simulink model "gm_DUALportRAMinterface_v3_vnl"  (R2024a)
settings: Solver=FixedStepDiscrete  StartTime=0.0  StopTime=0.1  RelTol=1e-3
undefined symbols (not defined in the file or in its folder): magnitude, Ts
libraries: hdlsllib x227, embmathops x6, simulink x2, hdlmdlgenlib x1, dsphdlxfrm2 x1
(part 5 of 6)

== system gm_DUALportRAMinterface_v3_vnl/PL/integration_block1/accumulator_scorer/64bitmsb_finder/8bit_PE7 ==
  D7 : Inport
  D6 : Inport  Port=2
  D5 : Inport  Port=3
  D4 : Inport  Port=4
  D3 : Inport  Port=5
  D2 : Inport  Port=6
  D1 : Inport  Port=7
  D0 : Inport  Port=8
  Add : Sum
  Bit Concat : hdlsllib/Logic and Bit Operations/Bit Concat  numInputs=3
  Constant2 : Constant  OutDataTypeStr=fixdt(0,4,0)  SampleTime=Ts
  Constant3 : Constant  Value=0  OutDataTypeStr=fixdt(0,4,0)  SampleTime=Ts
  Logical Operator{,10..16,22} (9 alike) : Logic  Operator=NOT  IconShape=distinctive  AllPortsSameDT=off  OutDataTypeStr=boolean
  Logical Operator1 : Logic  Operator=NAND  IconShape=distinctive  AllPortsSameDT=off  OutDataTypeStr=boolean
  Logical Operator{17..20} (4 alike) : Logic  Operator=OR  Inputs=4  IconShape=distinctive  AllPortsSameDT=off  OutDataTypeStr=boolean
  Logical Operator2 : Logic  Operator=NAND  Inputs=4  IconShape=distinctive  AllPortsSameDT=off  OutDataTypeStr=boolean
  Logical Operator21 : Logic  Operator=NAND  Inputs=3  IconShape=distinctive  AllPortsSameDT=off  OutDataTypeStr=boolean
  Logical Operator23 : Logic  IconShape=distinctive  AllPortsSameDT=off  OutDataTypeStr=boolean
  Logical Operator3 : Logic  Operator=NAND  Inputs=3  IconShape=distinctive  AllPortsSameDT=off  OutDataTypeStr=boolean
  Logical Operator4 : Logic  Inputs=3  IconShape=distinctive  AllPortsSameDT=off  OutDataTypeStr=boolean
  Logical Operator5 : Logic  Inputs=3  IconShape=distinctive  AllPortsSameDT=off  OutDataTypeStr=boolean
  Logical Operator6 : Logic  Inputs=4  IconShape=distinctive  AllPortsSameDT=off  OutDataTypeStr=boolean
  Logical Operator7 : Logic  Operator=NAND  Inputs=3  IconShape=distinctive  AllPortsSameDT=off  OutDataTypeStr=boolean
  Logical Operator8 : Logic  Operator=NAND  Inputs=4  IconShape=distinctive  AllPortsSameDT=off  OutDataTypeStr=boolean
  Logical Operator9 : Logic  Operator=NAND  Inputs=4  IconShape=distinctive  AllPortsSameDT=off  OutDataTypeStr=boolean
  Switch : Switch  Criteria=u2 > Threshold  SaturateOnIntegerOverflow=off  InputSameDT=off  OutDataTypeStr=Inherit: Same as first input
  data2 : Outport
  valid : Outport  Port=2
  wires:
  Logical Operator1/1 -> Logical Operator4/2, Logical Operator6/2, Logical Operator5/2, Logical Operator2/2, Logical Operator3/1, Logical Operator11/1
  Logical Operator2/1 -> Logical Operator6/4, Logical Operator8/2, Logical Operator7/2, Logical Operator13/1
  Logical Operator18/1 -> Bit Concat/2, Logical Operator20/3, Logical Operator21/2
  Logical Operator3/1 -> Logical Operator2/1, Logical Operator6/1, Logical Operator5/1, Logical Operator4/1, Logical Operator12/1
  Logical Operator13/1 -> Logical Operator17/4
  D4/1 -> Logical Operator2/4
  Logical Operator7/1 -> Logical Operator9/2, Logical Operator8/3, Logical Operator14/1
  Logical Operator/1 -> Logical Operator1/1, Logical Operator2/3, Logical Operator6/3, Logical Operator5/3, Logical Operator4/3, Logical Operator3/2, Logical Operator10/1
  Logical Operator12/1 -> Logical Operator17/3, Logical Operator19/2
  Logical Operator19/1 -> Logical Operator20/4, Logical Operator21/3, Bit Concat/3
  D3/1 -> Logical Operator7/3
  D7/1 -> Logical Operator/1
  Logical Operator15/1 -> Logical Operator18/4
  Logical Operator10/1 -> Logical Operator19/1, Logical Operator18/1, Logical Operator17/1
  Logical Operator14/1 -> Logical Operator18/3, Logical Operator19/4
  D5/1 -> Logical Operator3/3
  Logical Operator17/1 -> Logical Operator20/1, Logical Operator21/1, Bit Concat/1
  D2/1 -> Logical Operator8/4
  Logical Operator5/1 -> Logical Operator8/1
  D1/1 -> Logical Operator9/4
  Logical Operator4/1 -> Logical Operator7/1
  Logical Operator8/1 -> Logical Operator9/3, Logical Operator15/1
  Logical Operator6/1 -> Logical Operator9/1
  D6/1 -> Logical Operator1/2
  Logical Operator11/1 -> Logical Operator18/2, Logical Operator17/2
  Logical Operator16/1 -> Logical Operator19/3
  Logical Operator9/1 -> Logical Operator16/1
  D0/1 -> Logical Operator20/2
  Logical Operator20/1 -> valid/1, Logical Operator22/1
  Switch/1 -> Add/1
  Constant3/1 -> Switch/1
  Add/1 -> data2/1
  Bit Concat/1 -> Add/2
  Constant2/1 -> Switch/3
  Logical Operator21/1 -> Logical Operator23/1
  Logical Operator23/1 -> Switch/2
  Logical Operator22/1 -> Logical Operator23/2

== system gm_DUALportRAMinterface_v3_vnl/PL/integration_block1/accumulator_scorer/64bitmsb_finder/8bit_PE8 ==
  D7 : Inport
  D6 : Inport  Port=2
  D5 : Inport  Port=3
  D4 : Inport  Port=4
  D3 : Inport  Port=5
  D2 : Inport  Port=6
  D1 : Inport  Port=7
  D0 : Inport  Port=8
  Add : Sum
  Bit Concat : hdlsllib/Logic and Bit Operations/Bit Concat  numInputs=3
  Constant2 : Constant  OutDataTypeStr=fixdt(0,4,0)  SampleTime=Ts
  Constant3 : Constant  Value=0  OutDataTypeStr=fixdt(0,4,0)  SampleTime=Ts
  Logical Operator{,10..16,22} (9 alike) : Logic  Operator=NOT  IconShape=distinctive  AllPortsSameDT=off  OutDataTypeStr=boolean
  Logical Operator1 : Logic  Operator=NAND  IconShape=distinctive  AllPortsSameDT=off  OutDataTypeStr=boolean
  Logical Operator{17..20} (4 alike) : Logic  Operator=OR  Inputs=4  IconShape=distinctive  AllPortsSameDT=off  OutDataTypeStr=boolean
  Logical Operator2 : Logic  Operator=NAND  Inputs=4  IconShape=distinctive  AllPortsSameDT=off  OutDataTypeStr=boolean
  Logical Operator21 : Logic  Operator=NAND  Inputs=3  IconShape=distinctive  AllPortsSameDT=off  OutDataTypeStr=boolean
  Logical Operator23 : Logic  IconShape=distinctive  AllPortsSameDT=off  OutDataTypeStr=boolean
  Logical Operator3 : Logic  Operator=NAND  Inputs=3  IconShape=distinctive  AllPortsSameDT=off  OutDataTypeStr=boolean
  Logical Operator4 : Logic  Inputs=3  IconShape=distinctive  AllPortsSameDT=off  OutDataTypeStr=boolean
  Logical Operator5 : Logic  Inputs=3  IconShape=distinctive  AllPortsSameDT=off  OutDataTypeStr=boolean
  Logical Operator6 : Logic  Inputs=4  IconShape=distinctive  AllPortsSameDT=off  OutDataTypeStr=boolean
  Logical Operator7 : Logic  Operator=NAND  Inputs=3  IconShape=distinctive  AllPortsSameDT=off  OutDataTypeStr=boolean
  Logical Operator8 : Logic  Operator=NAND  Inputs=4  IconShape=distinctive  AllPortsSameDT=off  OutDataTypeStr=boolean
  Logical Operator9 : Logic  Operator=NAND  Inputs=4  IconShape=distinctive  AllPortsSameDT=off  OutDataTypeStr=boolean
  Switch : Switch  Criteria=u2 > Threshold  SaturateOnIntegerOverflow=off  InputSameDT=off  OutDataTypeStr=Inherit: Same as first input
  data2 : Outport
  valid : Outport  Port=2
  wires:
  Logical Operator22/1 -> Logical Operator23/2
  Logical Operator23/1 -> Switch/2
  Logical Operator21/1 -> Logical Operator23/1
  Constant2/1 -> Switch/3
  Bit Concat/1 -> Add/2
  Add/1 -> data2/1
  Constant3/1 -> Switch/1
  Switch/1 -> Add/1
  Logical Operator20/1 -> Logical Operator22/1, valid/1
  D0/1 -> Logical Operator20/2
  Logical Operator9/1 -> Logical Operator16/1
  Logical Operator16/1 -> Logical Operator19/3
  Logical Operator11/1 -> Logical Operator17/2, Logical Operator18/2
  D6/1 -> Logical Operator1/2
  Logical Operator6/1 -> Logical Operator9/1
  Logical Operator8/1 -> Logical Operator15/1, Logical Operator9/3
  Logical Operator4/1 -> Logical Operator7/1
  D1/1 -> Logical Operator9/4
  Logical Operator5/1 -> Logical Operator8/1
  D2/1 -> Logical Operator8/4
  Logical Operator17/1 -> Bit Concat/1, Logical Operator21/1, Logical Operator20/1
  D5/1 -> Logical Operator3/3
  Logical Operator14/1 -> Logical Operator19/4, Logical Operator18/3
  Logical Operator10/1 -> Logical Operator17/1, Logical Operator18/1, Logical Operator19/1
  Logical Operator15/1 -> Logical Operator18/4
  D7/1 -> Logical Operator/1
  D3/1 -> Logical Operator7/3
  Logical Operator19/1 -> Bit Concat/3, Logical Operator21/3, Logical Operator20/4
  Logical Operator12/1 -> Logical Operator19/2, Logical Operator17/3
  Logical Operator/1 -> Logical Operator10/1, Logical Operator3/2, Logical Operator4/3, Logical Operator5/3, Logical Operator6/3, Logical Operator2/3, Logical Operator1/1
  Logical Operator7/1 -> Logical Operator14/1, Logical Operator8/3, Logical Operator9/2
  D4/1 -> Logical Operator2/4
  Logical Operator13/1 -> Logical Operator17/4
  Logical Operator3/1 -> Logical Operator12/1, Logical Operator4/1, Logical Operator5/1, Logical Operator6/1, Logical Operator2/1
  Logical Operator18/1 -> Logical Operator21/2, Logical Operator20/3, Bit Concat/2
  Logical Operator2/1 -> Logical Operator13/1, Logical Operator7/2, Logical Operator8/2, Logical Operator6/4
  Logical Operator1/1 -> Logical Operator11/1, Logical Operator3/1, Logical Operator2/2, Logical Operator5/2, Logical Operator6/2, Logical Operator4/2

== system gm_DUALportRAMinterface_v3_vnl/PL/integration_block1/GA_main/coefficent_array/individual1/Subsystem ==
  reg_in : Inport
  enable : Inport  Port=2
  Delay : Delay  DelayLength=1  InitialCondition=0  SampleTime=Ts
  Switch : Switch  Criteria=u2 > Threshold  SaturateOnIntegerOverflow=off  InputSameDT=off
  reg_out : Outport
  wires:
  reg_in/1 -> Switch/1
  enable/1 -> Switch/2
  Switch/1 -> Delay/1
  Delay/1 -> Switch/3, reg_out/1

== system gm_DUALportRAMinterface_v3_vnl/PL/integration_block1/GA_main/coefficent_array/individual1/Subsystem1 ==
  reg_in : Inport
  enable : Inport  Port=2
  Delay : Delay  DelayLength=1  InitialCondition=0  SampleTime=Ts
  Switch : Switch  Criteria=u2 > Threshold  SaturateOnIntegerOverflow=off  InputSameDT=off
  reg_out : Outport
  wires:
  reg_in/1 -> Switch/1
  enable/1 -> Switch/2
  Switch/1 -> Delay/1
  Delay/1 -> Switch/3, reg_out/1

== system gm_DUALportRAMinterface_v3_vnl/PL/integration_block1/GA_main/coefficent_array/individual1/Subsystem2 ==
  reg_in : Inport
  enable : Inport  Port=2
  Delay : Delay  DelayLength=1  InitialCondition=0  SampleTime=Ts
  Switch : Switch  Criteria=u2 > Threshold  SaturateOnIntegerOverflow=off  InputSameDT=off
  reg_out : Outport
  wires:
  reg_in/1 -> Switch/1
  enable/1 -> Switch/2
  Switch/1 -> Delay/1
  Delay/1 -> Switch/3, reg_out/1

== system gm_DUALportRAMinterface_v3_vnl/PL/integration_block1/GA_main/coefficent_array/individual1/Subsystem3 ==
  reg_in : Inport
  enable : Inport  Port=2
  Delay : Delay  DelayLength=1  InitialCondition=0  SampleTime=Ts
  Switch : Switch  Criteria=u2 > Threshold  SaturateOnIntegerOverflow=off  InputSameDT=off
  reg_out : Outport
  wires:
  reg_in/1 -> Switch/1
  enable/1 -> Switch/2
  Switch/1 -> Delay/1
  Delay/1 -> Switch/3, reg_out/1

== system gm_DUALportRAMinterface_v3_vnl/PL/integration_block1/GA_main/coefficent_array/individual1/Subsystem4 ==
  reg_in : Inport
  enable : Inport  Port=2
  Delay : Delay  DelayLength=1  InitialCondition=0  SampleTime=Ts
  Switch : Switch  Criteria=u2 > Threshold  SaturateOnIntegerOverflow=off  InputSameDT=off
  reg_out : Outport
  wires:
  reg_in/1 -> Switch/1
  enable/1 -> Switch/2
  Switch/1 -> Delay/1
  Delay/1 -> Switch/3, reg_out/1

== system gm_DUALportRAMinterface_v3_vnl/PL/integration_block1/GA_main/coefficent_array/individual1/Subsystem5 ==
  reg_in : Inport
  enable : Inport  Port=2
  Delay : Delay  DelayLength=1  InitialCondition=0  SampleTime=Ts
  Switch : Switch  Criteria=u2 > Threshold  SaturateOnIntegerOverflow=off  InputSameDT=off
  reg_out : Outport
  wires:
  reg_in/1 -> Switch/1
  enable/1 -> Switch/2
  Switch/1 -> Delay/1
  Delay/1 -> Switch/3, reg_out/1

== system gm_DUALportRAMinterface_v3_vnl/PL/integration_block1/GA_main/coefficent_array/individual1/Subsystem6 ==
  reg_in : Inport
  enable : Inport  Port=2
  Delay : Delay  DelayLength=1  InitialCondition=0  SampleTime=Ts
  Switch : Switch  Criteria=u2 > Threshold  SaturateOnIntegerOverflow=off  InputSameDT=off
  reg_out : Outport
  wires:
  Delay/1 -> reg_out/1, Switch/3
  Switch/1 -> Delay/1
  enable/1 -> Switch/2
  reg_in/1 -> Switch/1

== system gm_DUALportRAMinterface_v3_vnl/PL/integration_block1/GA_main/coefficent_array/individual2/Subsystem ==
  reg_in : Inport
  enable : Inport  Port=2
  Delay : Delay  DelayLength=1  InitialCondition=0  SampleTime=Ts
  Switch : Switch  Criteria=u2 > Threshold  SaturateOnIntegerOverflow=off  InputSameDT=off
  reg_out : Outport
  wires:
  Delay/1 -> reg_out/1, Switch/3
  Switch/1 -> Delay/1
  enable/1 -> Switch/2
  reg_in/1 -> Switch/1

== system gm_DUALportRAMinterface_v3_vnl/PL/integration_block1/GA_main/coefficent_array/individual2/Subsystem1 ==
  reg_in : Inport
  enable : Inport  Port=2
  Delay : Delay  DelayLength=1  InitialCondition=0  SampleTime=Ts
  Switch : Switch  Criteria=u2 > Threshold  SaturateOnIntegerOverflow=off  InputSameDT=off
  reg_out : Outport
  wires:
  Delay/1 -> reg_out/1, Switch/3
  Switch/1 -> Delay/1
  enable/1 -> Switch/2
  reg_in/1 -> Switch/1

== system gm_DUALportRAMinterface_v3_vnl/PL/integration_block1/GA_main/coefficent_array/individual2/Subsystem2 ==
  reg_in : Inport
  enable : Inport  Port=2
  Delay : Delay  DelayLength=1  InitialCondition=0  SampleTime=Ts
  Switch : Switch  Criteria=u2 > Threshold  SaturateOnIntegerOverflow=off  InputSameDT=off
  reg_out : Outport
  wires:
  Delay/1 -> reg_out/1, Switch/3
  Switch/1 -> Delay/1
  enable/1 -> Switch/2
  reg_in/1 -> Switch/1

== system gm_DUALportRAMinterface_v3_vnl/PL/integration_block1/GA_main/coefficent_array/individual2/Subsystem3 ==
  reg_in : Inport
  enable : Inport  Port=2
  Delay : Delay  DelayLength=1  InitialCondition=0  SampleTime=Ts
  Switch : Switch  Criteria=u2 > Threshold  SaturateOnIntegerOverflow=off  InputSameDT=off
  reg_out : Outport
  wires:
  Delay/1 -> reg_out/1, Switch/3
  Switch/1 -> Delay/1
  enable/1 -> Switch/2
  reg_in/1 -> Switch/1

== system gm_DUALportRAMinterface_v3_vnl/PL/integration_block1/GA_main/coefficent_array/individual2/Subsystem4 ==
  reg_in : Inport
  enable : Inport  Port=2
  Delay : Delay  DelayLength=1  InitialCondition=0  SampleTime=Ts
  Switch : Switch  Criteria=u2 > Threshold  SaturateOnIntegerOverflow=off  InputSameDT=off
  reg_out : Outport
  wires:
  Delay/1 -> reg_out/1, Switch/3
  Switch/1 -> Delay/1
  enable/1 -> Switch/2
  reg_in/1 -> Switch/1

== system gm_DUALportRAMinterface_v3_vnl/PL/integration_block1/GA_main/coefficent_array/individual2/Subsystem5 ==
  reg_in : Inport
  enable : Inport  Port=2
  Delay : Delay  DelayLength=1  InitialCondition=0  SampleTime=Ts
  Switch : Switch  Criteria=u2 > Threshold  SaturateOnIntegerOverflow=off  InputSameDT=off
  reg_out : Outport
  wires:
  Delay/1 -> reg_out/1, Switch/3
  Switch/1 -> Delay/1
  enable/1 -> Switch/2
  reg_in/1 -> Switch/1

== system gm_DUALportRAMinterface_v3_vnl/PL/integration_block1/GA_main/coefficent_array/individual2/Subsystem6 ==
  reg_in : Inport
  enable : Inport  Port=2
  Delay : Delay  DelayLength=1  InitialCondition=0  SampleTime=Ts
  Switch : Switch  Criteria=u2 > Threshold  SaturateOnIntegerOverflow=off  InputSameDT=off
  reg_out : Outport
  wires:
  reg_in/1 -> Switch/1
  enable/1 -> Switch/2
  Switch/1 -> Delay/1
  Delay/1 -> Switch/3, reg_out/1

== system gm_DUALportRAMinterface_v3_vnl/PL/integration_block1/GA_main/coefficent_array/individual3/Subsystem ==
  reg_in : Inport
  enable : Inport  Port=2
  Delay : Delay  DelayLength=1  InitialCondition=0  SampleTime=Ts
  Switch : Switch  Criteria=u2 > Threshold  SaturateOnIntegerOverflow=off  InputSameDT=off
  reg_out : Outport
  wires:
  reg_in/1 -> Switch/1
  enable/1 -> Switch/2
  Switch/1 -> Delay/1
  Delay/1 -> Switch/3, reg_out/1

== system gm_DUALportRAMinterface_v3_vnl/PL/integration_block1/GA_main/coefficent_array/individual3/Subsystem1 ==
  reg_in : Inport
  enable : Inport  Port=2
  Delay : Delay  DelayLength=1  InitialCondition=0  SampleTime=Ts
  Switch : Switch  Criteria=u2 > Threshold  SaturateOnIntegerOverflow=off  InputSameDT=off
  reg_out : Outport
  wires:
  reg_in/1 -> Switch/1
  enable/1 -> Switch/2
  Switch/1 -> Delay/1
  Delay/1 -> Switch/3, reg_out/1

== system gm_DUALportRAMinterface_v3_vnl/PL/integration_block1/GA_main/coefficent_array/individual3/Subsystem2 ==
  reg_in : Inport
  enable : Inport  Port=2
  Delay : Delay  DelayLength=1  InitialCondition=0  SampleTime=Ts
  Switch : Switch  Criteria=u2 > Threshold  SaturateOnIntegerOverflow=off  InputSameDT=off
  reg_out : Outport
  wires:
  reg_in/1 -> Switch/1
  enable/1 -> Switch/2
  Switch/1 -> Delay/1
  Delay/1 -> Switch/3, reg_out/1

== system gm_DUALportRAMinterface_v3_vnl/PL/integration_block1/GA_main/coefficent_array/individual3/Subsystem3 ==
  reg_in : Inport
  enable : Inport  Port=2
  Delay : Delay  DelayLength=1  InitialCondition=0  SampleTime=Ts
  Switch : Switch  Criteria=u2 > Threshold  SaturateOnIntegerOverflow=off  InputSameDT=off
  reg_out : Outport
  wires:
  reg_in/1 -> Switch/1
  enable/1 -> Switch/2
  Switch/1 -> Delay/1
  Delay/1 -> Switch/3, reg_out/1

== system gm_DUALportRAMinterface_v3_vnl/PL/integration_block1/GA_main/coefficent_array/individual3/Subsystem4 ==
  reg_in : Inport
  enable : Inport  Port=2
  Delay : Delay  DelayLength=1  InitialCondition=0  SampleTime=Ts
  Switch : Switch  Criteria=u2 > Threshold  SaturateOnIntegerOverflow=off  InputSameDT=off
  reg_out : Outport
  wires:
  reg_in/1 -> Switch/1
  enable/1 -> Switch/2
  Switch/1 -> Delay/1
  Delay/1 -> Switch/3, reg_out/1

== system gm_DUALportRAMinterface_v3_vnl/PL/integration_block1/GA_main/coefficent_array/individual3/Subsystem5 ==
  reg_in : Inport
  enable : Inport  Port=2
  Delay : Delay  DelayLength=1  InitialCondition=0  SampleTime=Ts
  Switch : Switch  Criteria=u2 > Threshold  SaturateOnIntegerOverflow=off  InputSameDT=off
  reg_out : Outport
  wires:
  reg_in/1 -> Switch/1
  enable/1 -> Switch/2
  Switch/1 -> Delay/1
  Delay/1 -> Switch/3, reg_out/1

== system gm_DUALportRAMinterface_v3_vnl/PL/integration_block1/GA_main/coefficent_array/individual3/Subsystem6 ==
  reg_in : Inport
  enable : Inport  Port=2
  Delay : Delay  DelayLength=1  InitialCondition=0  SampleTime=Ts
  Switch : Switch  Criteria=u2 > Threshold  SaturateOnIntegerOverflow=off  InputSameDT=off
  reg_out : Outport
  wires:
  Delay/1 -> reg_out/1, Switch/3
  Switch/1 -> Delay/1
  enable/1 -> Switch/2
  reg_in/1 -> Switch/1

== system gm_DUALportRAMinterface_v3_vnl/PL/integration_block1/GA_main/coefficent_array/individual4/Subsystem ==
  reg_in : Inport
  enable : Inport  Port=2
  Delay : Delay  DelayLength=1  InitialCondition=0  SampleTime=Ts
  Switch : Switch  Criteria=u2 > Threshold  SaturateOnIntegerOverflow=off  InputSameDT=off
  reg_out : Outport
  wires:
  Delay/1 -> reg_out/1, Switch/3
  Switch/1 -> Delay/1
  enable/1 -> Switch/2
  reg_in/1 -> Switch/1

== system gm_DUALportRAMinterface_v3_vnl/PL/integration_block1/GA_main/coefficent_array/individual4/Subsystem1 ==
  reg_in : Inport
  enable : Inport  Port=2
  Delay : Delay  DelayLength=1  InitialCondition=0  SampleTime=Ts
  Switch : Switch  Criteria=u2 > Threshold  SaturateOnIntegerOverflow=off  InputSameDT=off
  reg_out : Outport
  wires:
  Delay/1 -> reg_out/1, Switch/3
  Switch/1 -> Delay/1
  enable/1 -> Switch/2
  reg_in/1 -> Switch/1

== system gm_DUALportRAMinterface_v3_vnl/PL/integration_block1/GA_main/coefficent_array/individual4/Subsystem2 ==
  reg_in : Inport
  enable : Inport  Port=2
  Delay : Delay  DelayLength=1  InitialCondition=0  SampleTime=Ts
  Switch : Switch  Criteria=u2 > Threshold  SaturateOnIntegerOverflow=off  InputSameDT=off
  reg_out : Outport
  wires:
  Delay/1 -> reg_out/1, Switch/3
  Switch/1 -> Delay/1
  enable/1 -> Switch/2
  reg_in/1 -> Switch/1

== system gm_DUALportRAMinterface_v3_vnl/PL/integration_block1/GA_main/coefficent_array/individual4/Subsystem3 ==
  reg_in : Inport
  enable : Inport  Port=2
  Delay : Delay  DelayLength=1  InitialCondition=0  SampleTime=Ts
  Switch : Switch  Criteria=u2 > Threshold  SaturateOnIntegerOverflow=off  InputSameDT=off
  reg_out : Outport
  wires:
  Delay/1 -> reg_out/1, Switch/3
  Switch/1 -> Delay/1
  enable/1 -> Switch/2
  reg_in/1 -> Switch/1

== system gm_DUALportRAMinterface_v3_vnl/PL/integration_block1/GA_main/coefficent_array/individual4/Subsystem4 ==
  reg_in : Inport
  enable : Inport  Port=2
  Delay : Delay  DelayLength=1  InitialCondition=0  SampleTime=Ts
  Switch : Switch  Criteria=u2 > Threshold  SaturateOnIntegerOverflow=off  InputSameDT=off
  reg_out : Outport
  wires:
  Delay/1 -> reg_out/1, Switch/3
  Switch/1 -> Delay/1
  enable/1 -> Switch/2
  reg_in/1 -> Switch/1

== system gm_DUALportRAMinterface_v3_vnl/PL/integration_block1/GA_main/coefficent_array/individual4/Subsystem5 ==
  reg_in : Inport
  enable : Inport  Port=2
  Delay : Delay  DelayLength=1  InitialCondition=0  SampleTime=Ts
  Switch : Switch  Criteria=u2 > Threshold  SaturateOnIntegerOverflow=off  InputSameDT=off
  reg_out : Outport
  wires:
  Delay/1 -> reg_out/1, Switch/3
  Switch/1 -> Delay/1
  enable/1 -> Switch/2
  reg_in/1 -> Switch/1

== system gm_DUALportRAMinterface_v3_vnl/PL/integration_block1/GA_main/coefficent_array/individual4/Subsystem6 ==
  reg_in : Inport
  enable : Inport  Port=2
  Delay : Delay  DelayLength=1  InitialCondition=0  SampleTime=Ts
  Switch : Switch  Criteria=u2 > Threshold  SaturateOnIntegerOverflow=off  InputSameDT=off
  reg_out : Outport
  wires:
  reg_in/1 -> Switch/1
  enable/1 -> Switch/2
  Switch/1 -> Delay/1
  Delay/1 -> Switch/3, reg_out/1

== system gm_DUALportRAMinterface_v3_vnl/PL/integration_block1/GA_main/coefficent_array1/individual1/Subsystem ==
  reg_in : Inport
  enable : Inport  Port=2
  Delay : Delay  DelayLength=1  InitialCondition=0  SampleTime=Ts
  Switch : Switch  Criteria=u2 > Threshold  SaturateOnIntegerOverflow=off  InputSameDT=off
  reg_out : Outport
  wires:
  Delay/1 -> reg_out/1, Switch/3
  Switch/1 -> Delay/1
  enable/1 -> Switch/2
  reg_in/1 -> Switch/1

== system gm_DUALportRAMinterface_v3_vnl/PL/integration_block1/GA_main/coefficent_array1/individual1/Subsystem1 ==
  reg_in : Inport
  enable : Inport  Port=2
  Delay : Delay  DelayLength=1  InitialCondition=0  SampleTime=Ts
  Switch : Switch  Criteria=u2 > Threshold  SaturateOnIntegerOverflow=off  InputSameDT=off
  reg_out : Outport
  wires:
  Delay/1 -> reg_out/1, Switch/3
  Switch/1 -> Delay/1
  enable/1 -> Switch/2
  reg_in/1 -> Switch/1

== system gm_DUALportRAMinterface_v3_vnl/PL/integration_block1/GA_main/coefficent_array1/individual1/Subsystem2 ==
  reg_in : Inport
  enable : Inport  Port=2
  Delay : Delay  DelayLength=1  InitialCondition=0  SampleTime=Ts
  Switch : Switch  Criteria=u2 > Threshold  SaturateOnIntegerOverflow=off  InputSameDT=off
  reg_out : Outport
  wires:
  Delay/1 -> reg_out/1, Switch/3
  Switch/1 -> Delay/1
  enable/1 -> Switch/2
  reg_in/1 -> Switch/1

== system gm_DUALportRAMinterface_v3_vnl/PL/integration_block1/GA_main/coefficent_array1/individual1/Subsystem3 ==
  reg_in : Inport
  enable : Inport  Port=2
  Delay : Delay  DelayLength=1  InitialCondition=0  SampleTime=Ts
  Switch : Switch  Criteria=u2 > Threshold  SaturateOnIntegerOverflow=off  InputSameDT=off
  reg_out : Outport
  wires:
  Delay/1 -> reg_out/1, Switch/3
  Switch/1 -> Delay/1
  enable/1 -> Switch/2
  reg_in/1 -> Switch/1

== system gm_DUALportRAMinterface_v3_vnl/PL/integration_block1/GA_main/coefficent_array1/individual1/Subsystem4 ==
  reg_in : Inport
  enable : Inport  Port=2
  Delay : Delay  DelayLength=1  InitialCondition=0  SampleTime=Ts
  Switch : Switch  Criteria=u2 > Threshold  SaturateOnIntegerOverflow=off  InputSameDT=off
  reg_out : Outport
  wires:
  Delay/1 -> reg_out/1, Switch/3
  Switch/1 -> Delay/1
  enable/1 -> Switch/2
  reg_in/1 -> Switch/1

== system gm_DUALportRAMinterface_v3_vnl/PL/integration_block1/GA_main/coefficent_array1/individual1/Subsystem5 ==
  reg_in : Inport
  enable : Inport  Port=2
  Delay : Delay  DelayLength=1  InitialCondition=0  SampleTime=Ts
  Switch : Switch  Criteria=u2 > Threshold  SaturateOnIntegerOverflow=off  InputSameDT=off
  reg_out : Outport
  wires:
  Delay/1 -> reg_out/1, Switch/3
  Switch/1 -> Delay/1
  enable/1 -> Switch/2
  reg_in/1 -> Switch/1

== system gm_DUALportRAMinterface_v3_vnl/PL/integration_block1/GA_main/coefficent_array1/individual1/Subsystem6 ==
  reg_in : Inport
  enable : Inport  Port=2
  Delay : Delay  DelayLength=1  InitialCondition=0  SampleTime=Ts
  Switch : Switch  Criteria=u2 > Threshold  SaturateOnIntegerOverflow=off  InputSameDT=off
  reg_out : Outport
  wires:
  reg_in/1 -> Switch/1
  enable/1 -> Switch/2
  Switch/1 -> Delay/1
  Delay/1 -> Switch/3, reg_out/1

== system gm_DUALportRAMinterface_v3_vnl/PL/integration_block1/GA_main/coefficent_array1/individual2/Subsystem ==
  reg_in : Inport
  enable : Inport  Port=2
  Delay : Delay  DelayLength=1  InitialCondition=0  SampleTime=Ts
  Switch : Switch  Criteria=u2 > Threshold  SaturateOnIntegerOverflow=off  InputSameDT=off
  reg_out : Outport
  wires:
  reg_in/1 -> Switch/1
  enable/1 -> Switch/2
  Switch/1 -> Delay/1
  Delay/1 -> Switch/3, reg_out/1

== system gm_DUALportRAMinterface_v3_vnl/PL/integration_block1/GA_main/coefficent_array1/individual2/Subsystem1 ==
  reg_in : Inport
  enable : Inport  Port=2
  Delay : Delay  DelayLength=1  InitialCondition=0  SampleTime=Ts
  Switch : Switch  Criteria=u2 > Threshold  SaturateOnIntegerOverflow=off  InputSameDT=off
  reg_out : Outport
  wires:
  reg_in/1 -> Switch/1
  enable/1 -> Switch/2
  Switch/1 -> Delay/1
  Delay/1 -> Switch/3, reg_out/1

== system gm_DUALportRAMinterface_v3_vnl/PL/integration_block1/GA_main/coefficent_array1/individual2/Subsystem2 ==
  reg_in : Inport
  enable : Inport  Port=2
  Delay : Delay  DelayLength=1  InitialCondition=0  SampleTime=Ts
  Switch : Switch  Criteria=u2 > Threshold  SaturateOnIntegerOverflow=off  InputSameDT=off
  reg_out : Outport
  wires:
  reg_in/1 -> Switch/1
  enable/1 -> Switch/2
  Switch/1 -> Delay/1
  Delay/1 -> Switch/3, reg_out/1

== system gm_DUALportRAMinterface_v3_vnl/PL/integration_block1/GA_main/coefficent_array1/individual2/Subsystem3 ==
  reg_in : Inport
  enable : Inport  Port=2
  Delay : Delay  DelayLength=1  InitialCondition=0  SampleTime=Ts
  Switch : Switch  Criteria=u2 > Threshold  SaturateOnIntegerOverflow=off  InputSameDT=off
  reg_out : Outport
  wires:
  reg_in/1 -> Switch/1
  enable/1 -> Switch/2
  Switch/1 -> Delay/1
  Delay/1 -> Switch/3, reg_out/1

== system gm_DUALportRAMinterface_v3_vnl/PL/integration_block1/GA_main/coefficent_array1/individual2/Subsystem4 ==
  reg_in : Inport
  enable : Inport  Port=2
  Delay : Delay  DelayLength=1  InitialCondition=0  SampleTime=Ts
  Switch : Switch  Criteria=u2 > Threshold  SaturateOnIntegerOverflow=off  InputSameDT=off
  reg_out : Outport
  wires:
  reg_in/1 -> Switch/1
  enable/1 -> Switch/2
  Switch/1 -> Delay/1
  Delay/1 -> Switch/3, reg_out/1

== system gm_DUALportRAMinterface_v3_vnl/PL/integration_block1/GA_main/coefficent_array1/individual2/Subsystem5 ==
  reg_in : Inport
  enable : Inport  Port=2
  Delay : Delay  DelayLength=1  InitialCondition=0  SampleTime=Ts
  Switch : Switch  Criteria=u2 > Threshold  SaturateOnIntegerOverflow=off  InputSameDT=off
  reg_out : Outport
  wires:
  reg_in/1 -> Switch/1
  enable/1 -> Switch/2
  Switch/1 -> Delay/1
  Delay/1 -> Switch/3, reg_out/1

== system gm_DUALportRAMinterface_v3_vnl/PL/integration_block1/GA_main/coefficent_array1/individual2/Subsystem6 ==
  reg_in : Inport
  enable : Inport  Port=2
  Delay : Delay  DelayLength=1  InitialCondition=0  SampleTime=Ts
  Switch : Switch  Criteria=u2 > Threshold  SaturateOnIntegerOverflow=off  InputSameDT=off
  reg_out : Outport
  wires:
  Delay/1 -> reg_out/1, Switch/3
  Switch/1 -> Delay/1
  enable/1 -> Switch/2
  reg_in/1 -> Switch/1

== system gm_DUALportRAMinterface_v3_vnl/PL/integration_block1/GA_main/coefficent_array1/individual3/Subsystem ==
  reg_in : Inport
  enable : Inport  Port=2
  Delay : Delay  DelayLength=1  InitialCondition=0  SampleTime=Ts
  Switch : Switch  Criteria=u2 > Threshold  SaturateOnIntegerOverflow=off  InputSameDT=off
  reg_out : Outport
  wires:
  Delay/1 -> reg_out/1, Switch/3
  Switch/1 -> Delay/1
  enable/1 -> Switch/2
  reg_in/1 -> Switch/1

== system gm_DUALportRAMinterface_v3_vnl/PL/integration_block1/GA_main/coefficent_array1/individual3/Subsystem1 ==
  reg_in : Inport
  enable : Inport  Port=2
  Delay : Delay  DelayLength=1  InitialCondition=0  SampleTime=Ts
  Switch : Switch  Criteria=u2 > Threshold  SaturateOnIntegerOverflow=off  InputSameDT=off
  reg_out : Outport
  wires:
  Delay/1 -> reg_out/1, Switch/3
  Switch/1 -> Delay/1
  enable/1 -> Switch/2
  reg_in/1 -> Switch/1

== system gm_DUALportRAMinterface_v3_vnl/PL/integration_block1/GA_main/coefficent_array1/individual3/Subsystem2 ==
  reg_in : Inport
  enable : Inport  Port=2
  Delay : Delay  DelayLength=1  InitialCondition=0  SampleTime=Ts
  Switch : Switch  Criteria=u2 > Threshold  SaturateOnIntegerOverflow=off  InputSameDT=off
  reg_out : Outport
  wires:
  Delay/1 -> reg_out/1, Switch/3
  Switch/1 -> Delay/1
  enable/1 -> Switch/2
  reg_in/1 -> Switch/1

== system gm_DUALportRAMinterface_v3_vnl/PL/integration_block1/GA_main/coefficent_array1/individual3/Subsystem3 ==
  reg_in : Inport
  enable : Inport  Port=2
  Delay : Delay  DelayLength=1  InitialCondition=0  SampleTime=Ts
  Switch : Switch  Criteria=u2 > Threshold  SaturateOnIntegerOverflow=off  InputSameDT=off
  reg_out : Outport
  wires:
  Delay/1 -> reg_out/1, Switch/3
  Switch/1 -> Delay/1
  enable/1 -> Switch/2
  reg_in/1 -> Switch/1

== system gm_DUALportRAMinterface_v3_vnl/PL/integration_block1/GA_main/coefficent_array1/individual3/Subsystem4 ==
  reg_in : Inport
  enable : Inport  Port=2
  Delay : Delay  DelayLength=1  InitialCondition=0  SampleTime=Ts
  Switch : Switch  Criteria=u2 > Threshold  SaturateOnIntegerOverflow=off  InputSameDT=off
  reg_out : Outport
  wires:
  Delay/1 -> reg_out/1, Switch/3
  Switch/1 -> Delay/1
  enable/1 -> Switch/2
  reg_in/1 -> Switch/1

== system gm_DUALportRAMinterface_v3_vnl/PL/integration_block1/GA_main/coefficent_array1/individual3/Subsystem5 ==
  reg_in : Inport
  enable : Inport  Port=2
  Delay : Delay  DelayLength=1  InitialCondition=0  SampleTime=Ts
  Switch : Switch  Criteria=u2 > Threshold  SaturateOnIntegerOverflow=off  InputSameDT=off
  reg_out : Outport
  wires:
  Delay/1 -> reg_out/1, Switch/3
  Switch/1 -> Delay/1
  enable/1 -> Switch/2
  reg_in/1 -> Switch/1

== system gm_DUALportRAMinterface_v3_vnl/PL/integration_block1/GA_main/coefficent_array1/individual3/Subsystem6 ==
  reg_in : Inport
  enable : Inport  Port=2
  Delay : Delay  DelayLength=1  InitialCondition=0  SampleTime=Ts
  Switch : Switch  Criteria=u2 > Threshold  SaturateOnIntegerOverflow=off  InputSameDT=off
  reg_out : Outport
  wires:
  reg_in/1 -> Switch/1
  enable/1 -> Switch/2
  Switch/1 -> Delay/1
  Delay/1 -> Switch/3, reg_out/1

== system gm_DUALportRAMinterface_v3_vnl/PL/integration_block1/GA_main/coefficent_array1/individual4/Subsystem ==
  reg_in : Inport
  enable : Inport  Port=2
  Delay : Delay  DelayLength=1  InitialCondition=0  SampleTime=Ts
  Switch : Switch  Criteria=u2 > Threshold  SaturateOnIntegerOverflow=off  InputSameDT=off
  reg_out : Outport
  wires:
  reg_in/1 -> Switch/1
  enable/1 -> Switch/2
  Switch/1 -> Delay/1
  Delay/1 -> Switch/3, reg_out/1

== system gm_DUALportRAMinterface_v3_vnl/PL/integration_block1/GA_main/coefficent_array1/individual4/Subsystem1 ==
  reg_in : Inport
  enable : Inport  Port=2
  Delay : Delay  DelayLength=1  InitialCondition=0  SampleTime=Ts
  Switch : Switch  Criteria=u2 > Threshold  SaturateOnIntegerOverflow=off  InputSameDT=off
  reg_out : Outport
  wires:
  reg_in/1 -> Switch/1
  enable/1 -> Switch/2
  Switch/1 -> Delay/1
  Delay/1 -> Switch/3, reg_out/1

== system gm_DUALportRAMinterface_v3_vnl/PL/integration_block1/GA_main/coefficent_array1/individual4/Subsystem2 ==
  reg_in : Inport
  enable : Inport  Port=2
  Delay : Delay  DelayLength=1  InitialCondition=0  SampleTime=Ts
  Switch : Switch  Criteria=u2 > Threshold  SaturateOnIntegerOverflow=off  InputSameDT=off
  reg_out : Outport
  wires:
  reg_in/1 -> Switch/1
  enable/1 -> Switch/2
  Switch/1 -> Delay/1
  Delay/1 -> Switch/3, reg_out/1

== system gm_DUALportRAMinterface_v3_vnl/PL/integration_block1/GA_main/coefficent_array1/individual4/Subsystem3 ==
  reg_in : Inport
  enable : Inport  Port=2
  Delay : Delay  DelayLength=1  InitialCondition=0  SampleTime=Ts
  Switch : Switch  Criteria=u2 > Threshold  SaturateOnIntegerOverflow=off  InputSameDT=off
  reg_out : Outport
  wires:
  reg_in/1 -> Switch/1
  enable/1 -> Switch/2
  Switch/1 -> Delay/1
  Delay/1 -> Switch/3, reg_out/1

== system gm_DUALportRAMinterface_v3_vnl/PL/integration_block1/GA_main/coefficent_array1/individual4/Subsystem4 ==
  reg_in : Inport
  enable : Inport  Port=2
  Delay : Delay  DelayLength=1  InitialCondition=0  SampleTime=Ts
  Switch : Switch  Criteria=u2 > Threshold  SaturateOnIntegerOverflow=off  InputSameDT=off
  reg_out : Outport
  wires:
  reg_in/1 -> Switch/1
  enable/1 -> Switch/2
  Switch/1 -> Delay/1
  Delay/1 -> Switch/3, reg_out/1

== system gm_DUALportRAMinterface_v3_vnl/PL/integration_block1/GA_main/coefficent_array1/individual4/Subsystem5 ==
  reg_in : Inport
  enable : Inport  Port=2
  Delay : Delay  DelayLength=1  InitialCondition=0  SampleTime=Ts
  Switch : Switch  Criteria=u2 > Threshold  SaturateOnIntegerOverflow=off  InputSameDT=off
  reg_out : Outport
  wires:
  reg_in/1 -> Switch/1
  enable/1 -> Switch/2
  Switch/1 -> Delay/1
  Delay/1 -> Switch/3, reg_out/1

== system gm_DUALportRAMinterface_v3_vnl/PL/integration_block1/GA_main/coefficent_array1/individual4/Subsystem6 ==
  reg_in : Inport
  enable : Inport  Port=2
  Delay : Delay  DelayLength=1  InitialCondition=0  SampleTime=Ts
  Switch : Switch  Criteria=u2 > Threshold  SaturateOnIntegerOverflow=off  InputSameDT=off
  reg_out : Outport
  wires:
  Delay/1 -> reg_out/1, Switch/3
  Switch/1 -> Delay/1
  enable/1 -> Switch/2
  reg_in/1 -> Switch/1

== stateflow chart gm_DUALportRAMinterface_v3_vnl/PL/integration_block1/FIFO_system1/Chart1 ==
  settings: updateMethod=DISCRETE  sampleTime=Ts  executeAtInitialization=1
  state initial_counter
    during:
    enable_counter = false;
  state counter_state
    during:
    enable_counter = true;
  (default) -> initial_counter
  counter_state -> initial_counter : [counter == 1+(4096+2048+1)]
  initial_counter -> counter_state : [en_out == true]
  data: counter input fixdt(0,13,0); enable_counter output boolean; en_out input boolean

== stateflow chart gm_DUALportRAMinterface_v3_vnl/PL/integration_block1/FIFO_system1/Chart2 ==
  settings: updateMethod=DISCRETE  sampleTime=Ts  executeAtInitialization=1
  state initial_push
    during:
    enable_push = false;
  state push_state
    during:
    enable_push = true;
  (default) -> initial_push
  push_state -> initial_push : [full == true]
  initial_push -> push_state : [load_FIFO1 == true]
  data: load_FIFO1 input boolean; full input boolean; enable_push output boolean

== stateflow chart gm_DUALportRAMinterface_v3_vnl/PL/Chart ==
  settings: executeAtInitialization=1
  state initial_wait_state
    entry:
    counter_increment = false;
    counter_reset = true;
    write_enable = false;
  state PL_read_data
    entry:
    counter_increment = true;
    counter_reset = false;
    write_enable = false;
  state wait_for_GA_done
    entry:
    counter_increment = false;
    counter_reset = true;
    write_enable = false;
  state reset_state
    entry:
    counter_increment = false;
    counter_reset = true;
    write_enable = false;
  state PL_write_data_back
    entry:
    counter_increment = true;
    counter_reset = false;
    write_enable = true;
  (default) -> initial_wait_state
  initial_wait_state -> PL_read_data : [GPIO == 1]
  PL_read_data -> wait_for_GA_done : [counter == (4096+2048+1)*2]
  wait_for_GA_done -> PL_write_data_back : [GA_done == 1]
  PL_write_data_back -> reset_state : [counter == 8]
  data: GA_done input boolean; GPIO input; counter input; counter_increment output boolean; counter_reset output boolean; write_enable output boolean

== stateflow chart gm_DUALportRAMinterface_v3_vnl/PL/integration_block1/FIFO_system1/Chart3 ==
  settings: updateMethod=DISCRETE  sampleTime=Ts  executeAtInitialization=1
  state initial_popstate
    during:
    enable_pop = false;
  state pop_state
    during:
    enable_pop = true;
  (default) -> initial_popstate
  pop_state -> initial_popstate : [counter == 2+(4096+2048+1)]
  initial_popstate -> pop_state : [counter == 1]
  data: enable_pop output boolean; counter input fixdt(0,13,0)

== stateflow chart gm_DUALportRAMinterface_v3_vnl/PL/integration_block1/FIFO_system3/Chart1 ==
  settings: updateMethod=DISCRETE  sampleTime=Ts  executeAtInitialization=1
  state initial_counter
    during:
    enable_counter = false;
  state counter_state
    during:
    enable_counter = true;
  (default) -> initial_counter
  counter_state -> initial_counter : [counter == 1+(4096+2048+1)]
  initial_counter -> counter_state : [en_out == true]
  data: counter input fixdt(0,13,0); enable_counter output boolean; en_out input boolean

== stateflow chart gm_DUALportRAMinterface_v3_vnl/PL/integration_block1/FIFO_system3/Chart2 ==
  settings: updateMethod=DISCRETE  sampleTime=Ts  executeAtInitialization=1
  state initial_push
    during:
    enable_push = false;
  state push_state
    during:
    enable_push = true;
  (default) -> initial_push
  push_state -> initial_push : [full == true]
  initial_push -> push_state : [load_FIFO1 == true]
  data: load_FIFO1 input boolean; full input boolean; enable_push output boolean

== stateflow chart gm_DUALportRAMinterface_v3_vnl/PL/integration_block1/FIFO_system3/Chart3 ==
  settings: updateMethod=DISCRETE  sampleTime=Ts  executeAtInitialization=1
  state initial_popstate
    during:
    enable_pop = false;
  state pop_state
    during:
    enable_pop = true;
  (default) -> initial_popstate
  pop_state -> initial_popstate : [counter == 2+(4096+2048+1)]
  initial_popstate -> pop_state : [counter == 1]
  data: enable_pop output boolean; counter input fixdt(0,13,0)

== stateflow chart gm_DUALportRAMinterface_v3_vnl/PL/integration_block1/GA_main/Chart ==
  settings: executeAtInitialization=1
  state index_and_hold
    entry:
    index_increment = true;
    slave_input = false;
    master_input = false;
    FIFO_out_en = false;
    exit:
    index_increment = false;
  state Enable_load_fifo
    load_fifo = true;
  state wait_for_FIFO
    load_fifo = false;
  state score_population
    entry:
    GA_done = false;
    a2_method = 1;
    a3_method = 1;
    a4_method = 1;
    b2_method = 1;
    b3_method = 1;
    b4_method = 1;
    slave_input = false;
    slave_output = true;
    master_input = true;
    master_output = 0;
    master_sort = false;
    generation_increment = false;
    generation_reset = false;
    index_increment = false;
    index_reset = false;
    FIFO_out_en = true;
  state initial_state
    during:
    GA_done = false;
    a2_method = 1;
    a3_method = 1;
    a4_method = 1;
    b2_method = 1;
    b3_method = 1;
    b4_method = 1;
    slave_input = false;
    slave_output = false;
    master_input = false;
    master_output = 0;
    master_sort = false;
    generation_increment = false;
    generation_reset = true;
    index_increment = false;
    index_reset = true;
    load_fifo = false;
    FIFO_out_en = false;
  state initial_random_population
    during:
    GA_done = false;
    a2_method = 1;
    a3_method = 1;
    a4_method = 1;
    b2_method = 1;
    b3_method = 1;
    b4_method = 1;
    slave_input = true;
    slave_output = false;
    master_input = false;
    master_output = 0;
    master_sort = false;
    generation_increment = false;
    generation_reset = false;
    index_increment = true;
    index_reset = false;
  state start_index_and_hold
    entry:
    index_reset = true;
    index_increment = true;
    slave_input = false;
    generation_increment = false;
    exit:
    index_increment = false;
    index_reset = false;
  state New_individual
    entry:
    a2_method = 1;
    a3_method = 1;
    a4_method = 1;
    b2_method = 1;
    b3_method = 1;
    b4_method = 1;
    slave_input = true;
    slave_output = false;
    master_input = false;
    master_output = 1;
    master_sort = false;
    generation_increment = false;
    generation_reset = false;
    index_increment = false;
    index_reset = false;
  state sort_population
    entry:
    slave_input = false;
    slave_output = false;
    master_input = false;
    master_output = 0;
    master_sort = true;
    generation_increment = false;
    generation_reset = false;
    index_increment = false;
    index_reset = true;
    FIFO_out_en = false;
  state Eliteism_or_Replication
    entry:
    a2_method = 3;
    a3_method = 3;
    a4_method = 3;
    b2_method = 3;
    b3_method = 3;
    b4_method = 3;
    slave_input = true;
    slave_output = false;
    master_input = false;
    master_output = 1;
    master_sort = false;
    generation_increment = false;
    generation_reset = false;
    index_increment = false;
    index_reset = false;
  state generation_update
    entry:
    slave_input = false;
    slave_output = false;
    master_input = false;
    master_output = 0;
    master_sort = false;
    generation_increment = true;
    generation_reset = false;
    index_increment = false;
    index_reset = true;
  state index_update
    entry:
    slave_input = false;
    slave_output = false;
    master_input = false;
    master_output = 0;
    master_sort = false;
    generation_increment = false;
    generation_reset = false;
    index_increment = true;
    index_reset = false;
  state GA_done_state
    entry:
    GA_done = true;
  state Crossover_load_dad
    entry:
    a2_method = 3;
    a3_method = 3;
    a4_method = 3;
    b2_method = 3;
    b3_method = 3;
    b4_method = 3;
    slave_input = false;
    slave_output = false;
    master_input = false;
    master_output = 2;
    master_sort = false;
    generation_increment = false;
    generation_reset = false;
    index_increment = false;
    index_reset = false;
  state Mutation1
    entry:
    a2_method = 1;
    a3_method = 3;
    a4_method = 3;
    b2_method = 3;
    b3_method = 3;
    b4_method = 3;
    slave_input = true;
    slave_output = false;
    master_input = false;
    master_output = 1;
    master_sort = false;
    generation_increment = false;
    generation_reset = false;
    index_increment = false;
    index_reset = false;
  state Mutation2
    entry:
    a2_method = 3;
    a3_method = 1;
    a4_method = 3;
    b2_method = 3;
    b3_method = 3;
    b4_method = 3;
    slave_input = true;
    slave_output = false;
    master_input = false;
    master_output = 1;
    master_sort = false;
    generation_increment = false;
    generation_reset = false;
    index_increment = false;
    index_reset = false;
  state Mutation3
    entry:
    a2_method = 3;
    a3_method = 3;
    a4_method = 1;
    b2_method = 3;
    b3_method = 3;
    b4_method = 3;
    slave_input = true;
    slave_output = false;
    master_input = false;
    master_output = 1;
    master_sort = false;
    generation_increment = false;
    generation_reset = false;
    index_increment = false;
    index_reset = false;
  state Mutation4
    entry:
    a2_method = 3;
    a3_method = 3;
    a4_method = 3;
    b2_method = 1;
    b3_method = 3;
    b4_method = 3;
    slave_input = true;
    slave_output = false;
    master_input = false;
    master_output = 1;
    master_sort = false;
    generation_increment = false;
    generation_reset = false;
    index_increment = false;
    index_reset = false;
  state Mutation5
    entry:
    a2_method = 3;
    a3_method = 3;
    a4_method = 3;
    b2_method = 3;
    b3_method = 1;
    b4_method = 3;
    slave_input = true;
    slave_output = false;
    master_input = false;
    master_output = 1;
    master_sort = false;
    generation_increment = false;
    generation_reset = false;
    index_increment = false;
    index_reset = false;
  state Mutation6
    entry:
    a2_method = 3;
    a3_method = 3;
    a4_method = 3;
    b2_method = 3;
    b3_method = 3;
    b4_method = 1;
    slave_input = true;
    slave_output = false;
    master_input = false;
    master_output = 1;
    master_sort = false;
    generation_increment = false;
    generation_reset = false;
    index_increment = false;
    index_reset = false;
  state Crossover1
    entry:
    a2_method = 2;
    a3_method = 3;
    a4_method = 3;
    b2_method = 3;
    b3_method = 3;
    b4_method = 3;
    slave_input = true;
    slave_output = false;
    master_input = false;
    master_output = 1;
    master_sort = false;
    generation_increment = false;
    generation_reset = false;
    index_increment = false;
    index_reset = false;
  state Crossover2
    entry:
    a2_method = 2;
    a3_method = 2;
    a4_method = 3;
    b2_method = 3;
    b3_method = 3;
    b4_method = 3;
    slave_input = true;
    slave_output = false;
    master_input = false;
    master_output = 1;
    master_sort = false;
    generation_increment = false;
    generation_reset = false;
    index_increment = false;
    index_reset = false;
  state Crossover3
    entry:
    a2_method = 2;
    a3_method = 2;
    a4_method = 2;
    b2_method = 3;
    b3_method = 3;
    b4_method = 3;
    slave_input = true;
    slave_output = false;
    master_input = false;
    master_output = 1;
    master_sort = false;
    generation_increment = false;
    generation_reset = false;
    index_increment = false;
    index_reset = false;
  state Crossover4
    entry:
    a2_method = 2;
    a3_method = 2;
    a4_method = 2;
    b2_method = 2;
    b3_method = 3;
    b4_method = 3;
    slave_input = true;
    slave_output = false;
    master_input = false;
    master_output = 1;
    master_sort = false;
    generation_increment = false;
    generation_reset = false;
    index_increment = false;
    index_reset = false;
  state Crossover5
    entry:
    a2_method = 2;
    a3_method = 2;
    a4_method = 2;
    b2_method = 2;
    b3_method = 2;
    b4_method = 3;
    slave_input = true;
    slave_output = false;
    master_input = false;
    master_output = 1;
    master_sort = false;
    generation_increment = false;
    generation_reset = false;
    index_increment = false;
    index_reset = false;
  Enable_load_fifo -> wait_for_FIFO
  score_population -> index_and_hold [order 2] : [score_done == 1]
  index_and_hold -> score_population
  (default) -> initial_state [order 1]
  initial_state -> Enable_load_fifo : [start_GA==1]
  wait_for_FIFO -> initial_random_population : [FIFO_full == 1]
  initial_random_population -> start_index_and_hold : [sample_index == 5]
  start_index_and_hold -> score_population
  generation_update -> start_index_and_hold [order 2]
  score_population -> sort_population [order 1] : [sample_index==4 & score_done==1]
  New_individual -> (junction 296)
  GA_done_state -> initial_state
  (junction 296) -> (junction 297)
  (junction 289) -> New_individual
  (junction 287) -> (junction 289) : [selected_method==4]
  sort_population -> index_update : [sort_done==1]
  (junction 297) -> index_update
  index_update -> (junction 287) [order 4]
  Eliteism_or_Replication -> index_update
  index_update -> Eliteism_or_Replication [order 2] : [sample_index==1 | selected_method==1]
  generation_update -> GA_done_state [order 1] : [generation_counter==10000]
  index_update -> generation_update [order 1] : [sample_index==5]
  (junction 221) -> index_update
  (junction 227) -> (junction 221)
  (junction 229) -> (junction 227)
  (junction 231) -> (junction 229)
  (junction 272) -> (junction 231)
  Mutation2 -> (junction 221)
  Mutation3 -> (junction 227)
  Mutation4 -> (junction 229)
  Mutation5 -> (junction 231)
  Mutation6 -> (junction 272)
  (junction 236) -> index_update
  Mutation1 -> index_update
  index_update -> (junction 175) [order 3] : [selected_method==2]
  (default) -> Crossover_load_dad [order 2] : [selected_method==3]
  (junction 175) -> (junction 177) [order 1]
  (junction 177) -> (junction 178) [order 1]
  (junction 178) -> (junction 179) [order 1]
  (junction 179) -> (junction 180) [order 1]
  (junction 180) -> (junction 267) [order 2]
  (junction 175) -> Mutation1 [order 2] : [random_gene==1]
  (junction 177) -> Mutation2 [order 2] : [random_gene==2]
  (junction 178) -> Mutation3 [order 2] : [random_gene==3]
  (junction 179) -> Mutation4 [order 2] : [random_gene==4]
  (junction 180) -> Mutation5 [order 1] : [random_gene==5]
  (junction 267) -> Mutation6 : [random_gene==6]
  Crossover_load_dad -> (junction 212)
  (junction 237) -> (junction 236)
  (junction 239) -> (junction 237)
  (junction 241) -> (junction 239)
  (junction 277) -> (junction 241)
  Crossover1 -> (junction 236)
  Crossover2 -> (junction 237)
  Crossover3 -> (junction 239)
  Crossover4 -> (junction 241)
  Crossover5 -> (junction 277)
  (junction 212) -> (junction 213) [order 1]
  (junction 213) -> (junction 203) [order 1]
  (junction 203) -> (junction 210) [order 1]
  (junction 210) -> (junction 271) [order 2]
  (junction 212) -> Crossover1 [order 2] : [random_gene==1]
  (junction 213) -> Crossover2 [order 2] : [random_gene==2]
  (junction 203) -> Crossover3 [order 2] : [random_gene==3]
  (junction 210) -> Crossover4 [order 1] : [random_gene==4]
  (junction 271) -> Crossover5 : [random_gene==5|random_gene==6]
  data: GA_done output boolean; index_reset output boolean; index_increment output boolean; a2_method output fixdt(0,2,0); a3_method output fixdt(0,2,0); a4_method output fixdt(0,2,0); b4_method output fixdt(0,2,0); b2_method output fixdt(0,2,0); b3_method output fixdt(0,2,0); sort_done input boolean; start_GA input boolean; score_done input boolean; FIFO_full input boolean; random_gene input fixdt(0,3,0); selected_method input fixdt(0,3,0); slave_input output boolean; slave_output output boolean; master_input output boolean; generation_increment output boolean; generation_reset output boolean; master_output output fixdt(0,2,0); master_sort output boolean; sample_index input fixdt(0,4,0); generation_counter input fixdt(0,16,0); FIFO_out_en output boolean; load_fifo output boolean
